simulink model "rw_torque"  (R2023b)
settings: Solver=VariableStepAuto  StartTime=0.0  StopTime=10.0  RelTol=1e-3
undefined symbols (not defined in the file or in its folder): sat
libraries: matrix_library x1
settings Model: Creator=aryam  LastModifiedBy=aryam

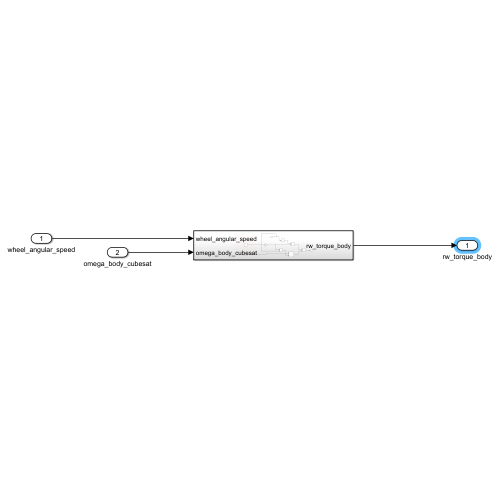
[thumbnail: Simulink's stored preview of the top-level diagram]
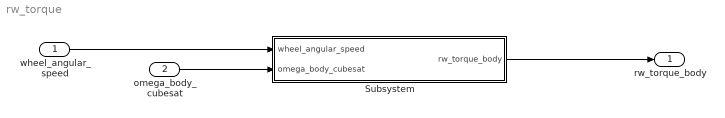
== system rw_torque ==
  wheel_angular_speed : Inport
  omega_body_cubesat : Inport  Port=2
  Subsystem : Subsystem
  rw_torque_body : Outport
  wires:
  wheel_angular_speed/1 -> Subsystem/1(wheel_angular_speed)
  omega_body_cubesat/1 -> Subsystem/2(omega_body_cubesat)
  Subsystem/1(rw_torque_body) -> rw_torque_body/1

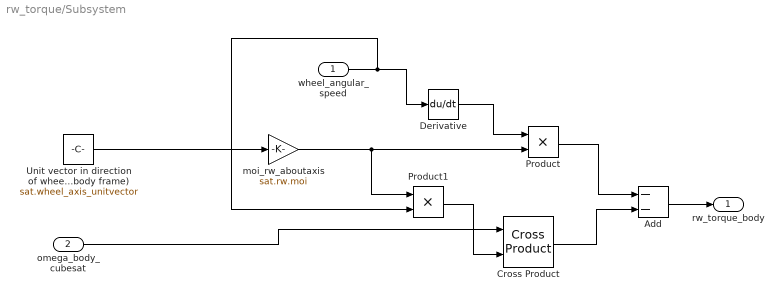
== system rw_torque/Subsystem ==
  wheel_angular_speed : Inport
  omega_body_cubesat : Inport  Port=2
  Add : Sum  Inputs=--
  Cross Product : matrix_library/Cross Product
  Derivative : Derivative
  Product : Product
  Product1 : Product
  "Unit vector in direction of wheel axis(here y-axis in body frame) " : Constant  Value=sat.wheel_axis_unitvector
  moi_rw_aboutaxis : Gain  Gain=sat.rw.moi
  rw_torque_body : Outport
  wires:
  Cross Product/1 -> Add/2
  wheel_angular_speed/1 -> Product1/2, Derivative/1
  "Unit vector in direction of wheel axis(here y-axis in body frame) "/1 -> moi_rw_aboutaxis/1
  moi_rw_aboutaxis/1 -> Product1/1, Product/2
  omega_body_cubesat/1 -> Cross Product/1
  Product1/1 -> Cross Product/2
  Product/1 -> Add/1
  Derivative/1 -> Product/1
  Add/1 -> rw_torque_body/1
